simulink library "propulsive"  (R2023a)
settings: Solver=VariableStepAuto  StartTime=0.0  StopTime=10.0  RelTol=1e-3
settings Model: Creator=User  LastModifiedBy=User

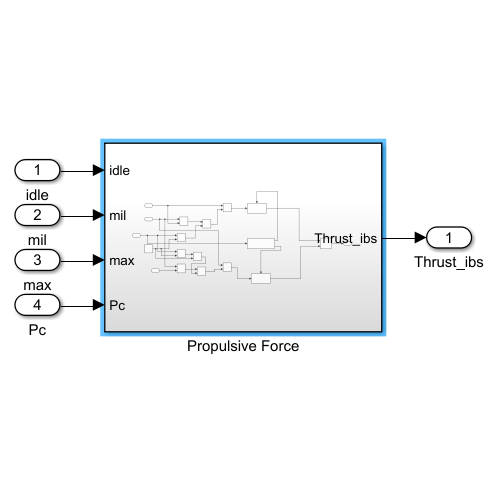
[thumbnail: Simulink's stored preview of the top-level diagram]
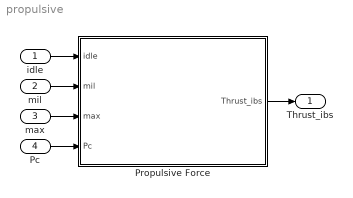
== system propulsive ==
  idle : Inport
  mil : Inport  Port=2
  max : Inport  Port=3
  Pc : Inport  Port=4
  Propulsive Force : Subsystem
  Thrust_ibs : Outport
  wires:
  idle/1 -> Propulsive Force/1(idle)
  mil/1 -> Propulsive Force/2(mil)
  max/1 -> Propulsive Force/3(max)
  Pc/1 -> Propulsive Force/4(Pc)
  Propulsive Force/1(Thrust_ibs) -> Thrust_ibs/1

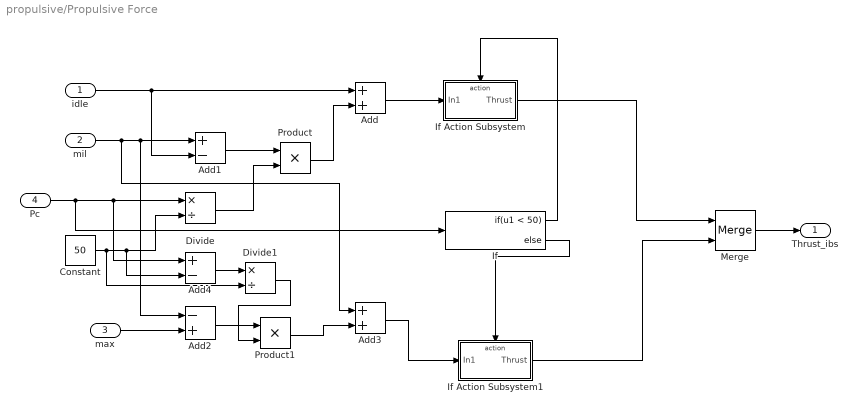
== system propulsive/Propulsive Force ==
  idle : Inport
  mil : Inport  Port=2
  max : Inport  Port=3
  Pc : Inport  Port=4
  Add : Sum
  Add1 : Sum  Inputs=+-
  Add2 : Sum  Inputs=-+
  Add3 : Sum
  Add4 : Sum  Inputs=+-
  Constant : Constant  Value=50
  Divide : Product  Inputs=*/
  Divide1 : Product  Inputs=*/
  If : If  IfExpression=u1 < 50
  If Action Subsystem : Subsystem  TreatAsAtomicUnit=on
  If Action Subsystem1 : Subsystem  TreatAsAtomicUnit=on
  Merge : Merge
  Product : Product
  Product1 : Product
  Thrust_ibs : Outport
  wires:
  Pc/1 -> If/1, Add4/1, Divide/1
  If/1 -> If Action Subsystem/Action
  max/1 -> Add2/2
  mil/1 -> Add2/1, Add1/1, Add3/1
  Constant/1 -> Divide1/2, Add4/2, Divide/2
  Divide/1 -> Product/2
  Product1/1 -> Add3/2
  idle/1 -> Add1/2, Add/1
  If Action Subsystem/1(Thrust) -> Merge/1
  Add2/1 -> Product1/1
  Add3/1 -> If Action Subsystem1/1(In1)
  Divide1/1 -> Product1/2
  Add4/1 -> Divide1/1
  Add1/1 -> Product/1
  Product/1 -> Add/2
  Add/1 -> If Action Subsystem/1(In1)
  If/2 -> If Action Subsystem1/Action
  If Action Subsystem1/1(Thrust) -> Merge/2
  Merge/1 -> Thrust_ibs/1

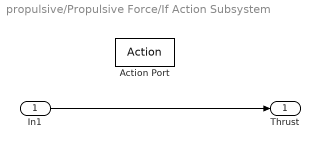
== system propulsive/Propulsive Force/If Action Subsystem ==
  In1 : Inport
  Action Port : ActionPort  ActionPortLabel=if(u1 < 50)
  Thrust : Outport
  wires:
  In1/1 -> Thrust/1

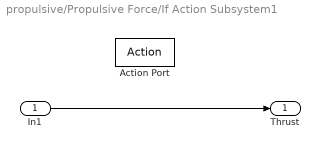
== system propulsive/Propulsive Force/If Action Subsystem1 ==
  In1 : Inport
  Action Port : ActionPort  ActionPortLabel=else
  Thrust : Outport
  wires:
  In1/1 -> Thrust/1
